simulink library "StIsPosChkLib"  (R2018b)
settings: Solver=VariableStepAuto  StartTime=0.0  StopTime=10.0  RelTol=1e-3
libraries: $bdroot x2, simulink x1
settings Model: Creator=sn2xws  LastModifiedBy=sn2xws

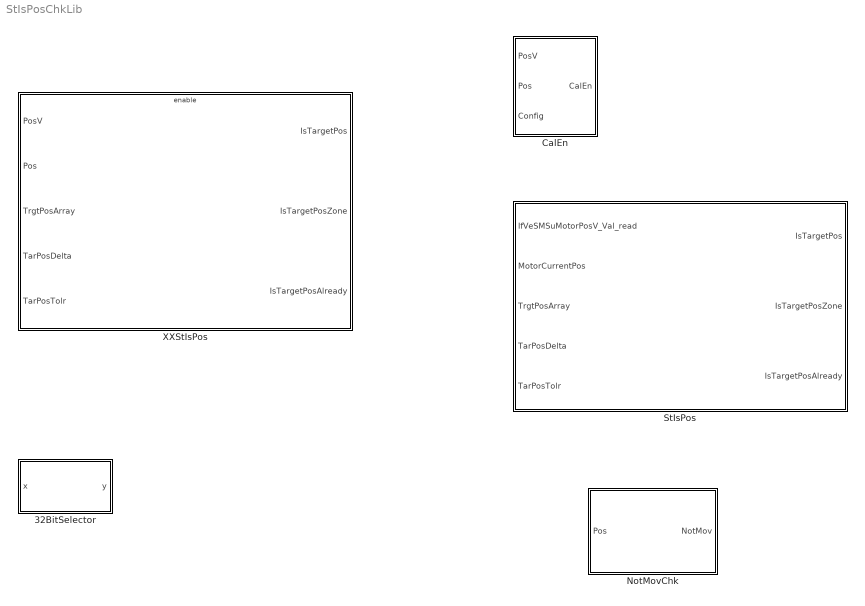
== system StIsPosChkLib ==
  32BitSelector : Subsystem  mask(32 Bit Selector){BitNum=1}
      mask prompts: BitNum "Select Bit Number"
      mask help: Allows selection of a particular bit (0-31) out of a packed word up to 32 bits long. Output will be true if the bit number selected via the mask parameter is equal to one.
      mask TypeOptions BitNum: 0 | 1 | 2 | 3 | 4 | 5 | 6 | 7 | 8 | 9 | 10 | 11 | 12 | 13 | 14 | 15 | 16 | 17 | 18 | 19 | 20 | 21 | 22 | 23 | 24 | 25 | 26 | 27 | 28 | 29 | 30 | 31
      mask Display:
      | text(0.5, 0.8,'BIT','horizontalAlignment','center')
      | text(0.5, 0.5,'SELECTOR','horizontalAlignment','center')
      | text(0.5, 0.2,['-- Bit ',char(get_param(gcb,'BitNum')),' --'],'horizontalAlignment','center')
  CalEn : Subsystem
  NotMovChk : Subsystem
  StIsPos : Subsystem
  XXStIsPos : Subsystem

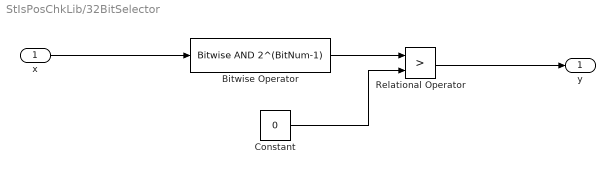
== system StIsPosChkLib/32BitSelector ==
  x : Inport
  Bitwise Operator : simulink/Logic and Bit Operations/Bitwise Operator  logicop=AND  UseBitMask=on  BitMask=2^(BitNum-1)  BitMaskRealWorld=Stored Integer
  Constant : Constant  Value=0  OutDataTypeStr=uint32
  Relational Operator : RelationalOperator  Operator=>  OutDataTypeStr=boolean  RndMeth=Simplest
  y : Outport
  wires:
  Bitwise Operator/1 -> Relational Operator/1
  x/1 -> Bitwise Operator/1
  Constant/1 -> Relational Operator/2
  Relational Operator/1 -> y/1

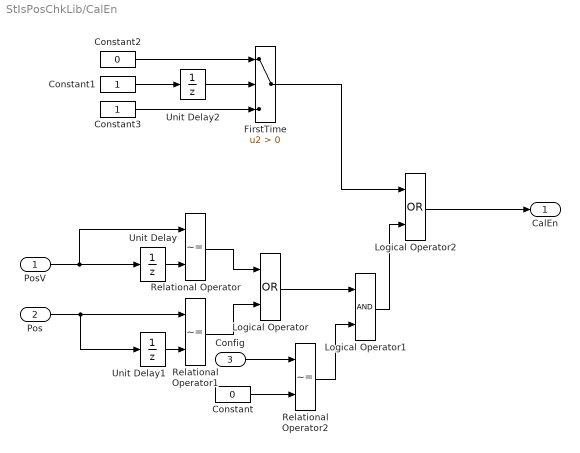
== system StIsPosChkLib/CalEn ==
  PosV : Inport
  Pos : Inport  Port=2
  Config : Inport  Port=3
  Constant : Constant  Value=0  OutDataTypeStr=uint8
  Constant1 : Constant  OutDataTypeStr=boolean
  Constant2 : Constant  Value=0  OutDataTypeStr=boolean
  Constant3 : Constant  OutDataTypeStr=boolean
  FirstTime : Switch  Criteria=u2 > Threshold
  Logical Operator : Logic  Operator=OR  AllPortsSameDT=off  OutDataTypeStr=boolean
  Logical Operator1 : Logic  AllPortsSameDT=off  OutDataTypeStr=boolean
  Logical Operator2 : Logic  Operator=OR  AllPortsSameDT=off  OutDataTypeStr=boolean
  Relational Operator : RelationalOperator  Operator=~=  OutDataTypeStr=boolean  RndMeth=Simplest
  Relational Operator1 : RelationalOperator  Operator=~=  OutDataTypeStr=boolean  RndMeth=Simplest
  Relational Operator2 : RelationalOperator  Operator=~=  OutDataTypeStr=boolean  RndMeth=Simplest
  Unit Delay : UnitDelay  SampleTime=-1
  Unit Delay1 : UnitDelay  SampleTime=-1
  Unit Delay2 : UnitDelay  SampleTime=-1
  CalEn : Outport
  wires:
  Logical Operator/1 -> Logical Operator1/1
  Relational Operator1/1 -> Logical Operator/2
  Unit Delay1/1 -> Relational Operator1/2
  Pos/1 -> Relational Operator1/1, Unit Delay1/1
  Relational Operator/1 -> Logical Operator/1
  Unit Delay/1 -> Relational Operator/2
  PosV/1 -> Unit Delay/1, Relational Operator/1
  Relational Operator2/1 -> Logical Operator1/2
  Config/1 -> Relational Operator2/1
  Constant/1 -> Relational Operator2/2
  Logical Operator1/1 -> Logical Operator2/2
  Logical Operator2/1 -> CalEn/1
  FirstTime/1 -> Logical Operator2/1
  Constant1/1 -> Unit Delay2/1
  Unit Delay2/1 -> FirstTime/2
  Constant2/1 -> FirstTime/1
  Constant3/1 -> FirstTime/3

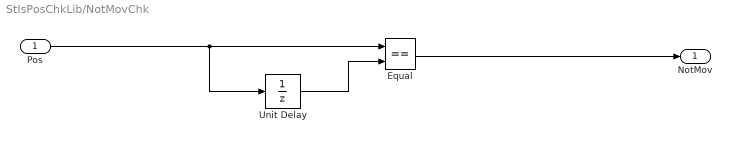
== system StIsPosChkLib/NotMovChk ==
  Pos : Inport
  Equal : RelationalOperator  Operator===  OutDataTypeStr=boolean  RndMeth=Simplest
  Unit Delay : UnitDelay  SampleTime=-1
  NotMov : Outport
  wires:
  Equal/1 -> NotMov/1
  Pos/1 -> Equal/1, Unit Delay/1
  Unit Delay/1 -> Equal/2

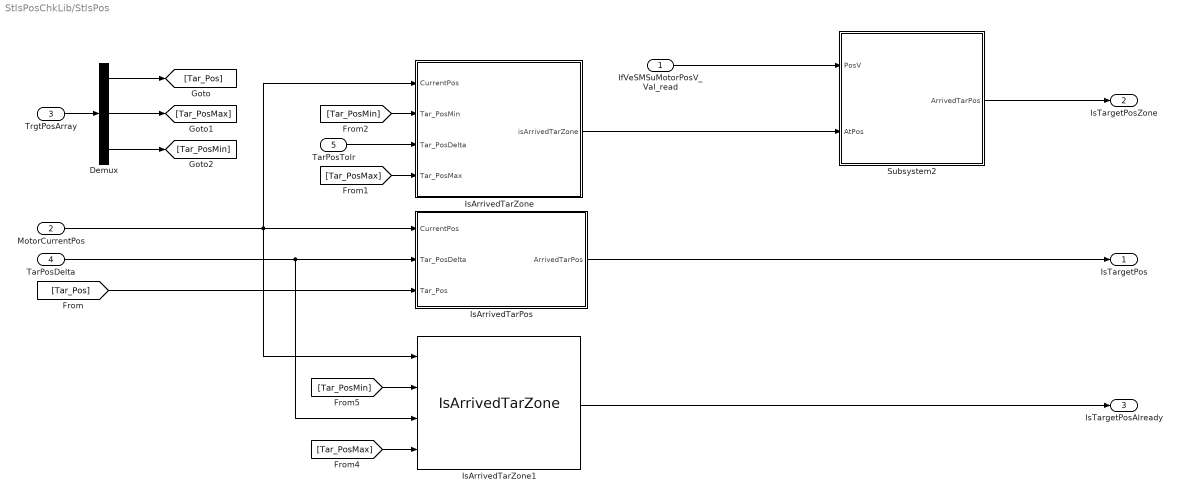
== system StIsPosChkLib/StIsPos ==
  IfVeSMSuMotorPosV_Val_read : Inport
  MotorCurrentPos : Inport  Port=2
  TrgtPosArray : Inport  Port=3
  TarPosDelta : Inport  Port=4
  TarPosTolr : Inport  Port=5
  Demux : Demux  Outputs=3
  IsArrivedTarPos : Subsystem
  IsArrivedTarZone : Subsystem
  IsArrivedTarZone1 : $bdroot/StIsPos/IsArrivedTarZone  SystemSampleTime=-1
  Subsystem2 : Subsystem
  IsTargetPos : Outport
      settings: EnsureOutportIsVirtual=on
  IsTargetPosZone : Outport  Port=2
      settings: EnsureOutportIsVirtual=on
  IsTargetPosAlready : Outport  Port=3
      settings: EnsureOutportIsVirtual=on
  wires:
  MotorCurrentPos/1 -> IsArrivedTarZone/1(CurrentPos), IsArrivedTarZone1/1, IsArrivedTarPos/1(CurrentPos)
  IsArrivedTarPos/1(ArrivedTarPos) -> IsTargetPos/1
  Subsystem2/1(ArrivedTarPos) -> IsTargetPosZone/1
  IfVeSMSuMotorPosV_Val_read/1 -> Subsystem2/1(PosV)
  IsArrivedTarZone/1(isArrivedTarZone) -> Subsystem2/2(AtPos)
  TrgtPosArray/1 -> Demux/1
  Demux/1 -> [Tar_Pos]
  Demux/2 -> [Tar_PosMax]
  Demux/3 -> [Tar_PosMin]
  [Tar_Pos] -> IsArrivedTarPos/3(Tar_Pos)
  [Tar_PosMax] -> IsArrivedTarZone/4(Tar_PosMax)
  [Tar_PosMin] -> IsArrivedTarZone/2(Tar_PosMin)
  [Tar_PosMax] -> IsArrivedTarZone1/4
  [Tar_PosMin] -> IsArrivedTarZone1/2
  TarPosDelta/1 -> IsArrivedTarZone1/3, IsArrivedTarPos/2(Tar_PosDelta)
  TarPosTolr/1 -> IsArrivedTarZone/3(Tar_PosDelta)
  IsArrivedTarZone1/1 -> IsTargetPosAlready/1

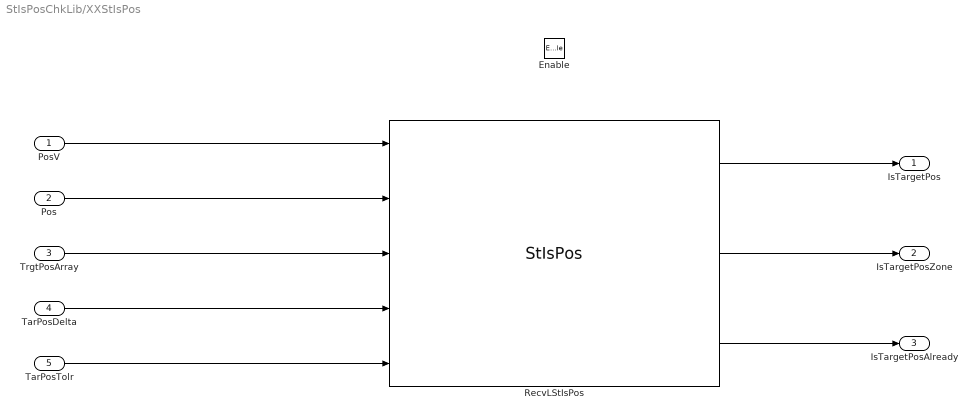
== system StIsPosChkLib/XXStIsPos ==
  PosV : Inport
  Pos : Inport  Port=2
  TrgtPosArray : Inport  Port=3
  TarPosDelta : Inport  Port=4
  TarPosTolr : Inport  Port=5
  Enable : EnablePort
  RecvLStIsPos : $bdroot/StIsPos  SystemSampleTime=-1
  IsTargetPos : Outport
  IsTargetPosZone : Outport  Port=2
  IsTargetPosAlready : Outport  Port=3
  wires:
  TarPosTolr/1 -> RecvLStIsPos/5
  TrgtPosArray/1 -> RecvLStIsPos/3
  PosV/1 -> RecvLStIsPos/1
  TarPosDelta/1 -> RecvLStIsPos/4
  Pos/1 -> RecvLStIsPos/2
  RecvLStIsPos/1 -> IsTargetPos/1
  RecvLStIsPos/3 -> IsTargetPosAlready/1
  RecvLStIsPos/2 -> IsTargetPosZone/1

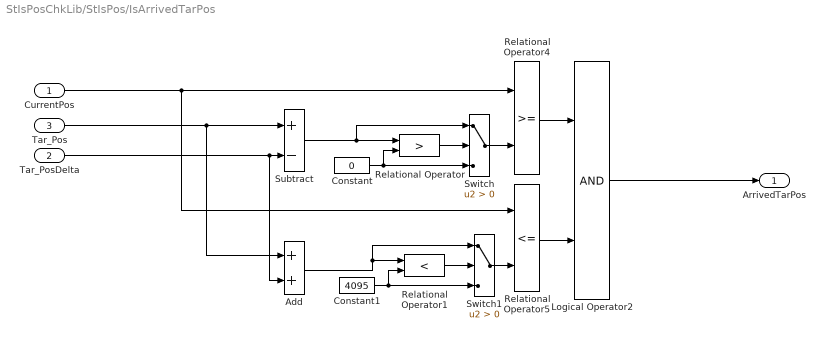
== system StIsPosChkLib/StIsPos/IsArrivedTarPos ==
  CurrentPos : Inport
  Tar_PosDelta : Inport  Port=2
  Tar_Pos : Inport  Port=3
  Add : Sum
  Constant : Constant  Value=0  OutDataTypeStr=uint16
  Constant1 : Constant  Value=4095  OutDataTypeStr=uint16
  Logical Operator2 : Logic  AllPortsSameDT=off  OutDataTypeStr=boolean
  Relational Operator : RelationalOperator  Operator=>  OutDataTypeStr=boolean  RndMeth=Simplest
  Relational Operator1 : RelationalOperator  Operator=<  OutDataTypeStr=boolean  RndMeth=Simplest
  Relational Operator4 : RelationalOperator  OutDataTypeStr=boolean  RndMeth=Simplest
  Relational Operator5 : RelationalOperator  Operator=<=  OutDataTypeStr=boolean  RndMeth=Simplest
  Subtract : Sum  Inputs=+-  OutDataTypeStr=int16
  Switch : Switch  Criteria=u2 > Threshold
  Switch1 : Switch  Criteria=u2 > Threshold
  ArrivedTarPos : Outport
  wires:
  Relational Operator5/1 -> Logical Operator2/2
  Tar_Pos/1 -> Add/1, Subtract/1
  Relational Operator4/1 -> Logical Operator2/1
  Tar_PosDelta/1 -> Add/2, Subtract/2
  Switch/1 -> Relational Operator4/2
  CurrentPos/1 -> Relational Operator4/1, Relational Operator5/1
  Logical Operator2/1 -> ArrivedTarPos/1
  Subtract/1 -> Switch/1, Relational Operator/1
  Relational Operator/1 -> Switch/2
  Constant/1 -> Relational Operator/2, Switch/3
  Add/1 -> Switch1/1, Relational Operator1/1
  Constant1/1 -> Relational Operator1/2, Switch1/3
  Switch1/1 -> Relational Operator5/2
  Relational Operator1/1 -> Switch1/2

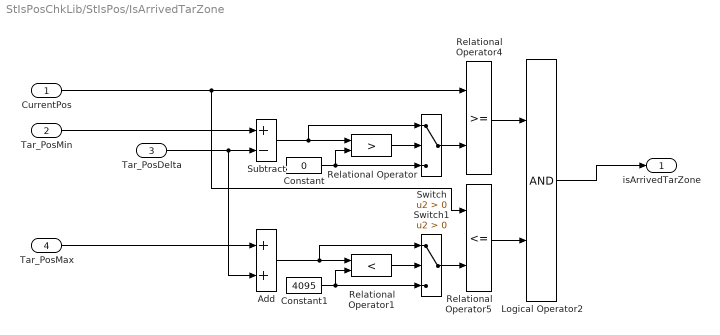
== system StIsPosChkLib/StIsPos/IsArrivedTarZone ==
  CurrentPos : Inport
  Tar_PosMin : Inport  Port=2
  Tar_PosDelta : Inport  Port=3
  Tar_PosMax : Inport  Port=4
  Add : Sum
  Constant : Constant  Value=0  OutDataTypeStr=uint16
  Constant1 : Constant  Value=4095  OutDataTypeStr=uint16
  Logical Operator2 : Logic  AllPortsSameDT=off  OutDataTypeStr=boolean
  Relational Operator : RelationalOperator  Operator=>  OutDataTypeStr=boolean  RndMeth=Simplest
  Relational Operator1 : RelationalOperator  Operator=<  OutDataTypeStr=boolean  RndMeth=Simplest
  Relational Operator4 : RelationalOperator  OutDataTypeStr=boolean  RndMeth=Simplest
  Relational Operator5 : RelationalOperator  Operator=<=  OutDataTypeStr=boolean  RndMeth=Simplest
  Subtract : Sum  Inputs=+-  OutDataTypeStr=int16
  Switch : Switch  Criteria=u2 > Threshold
  Switch1 : Switch  Criteria=u2 > Threshold
  isArrivedTarZone : Outport
  wires:
  Tar_PosDelta/1 -> Subtract/2, Add/2
  Add/1 -> Switch1/1, Relational Operator1/1
  Switch1/1 -> Relational Operator5/2
  CurrentPos/1 -> Relational Operator4/1, Relational Operator5/1
  Tar_PosMin/1 -> Subtract/1
  Switch/1 -> Relational Operator4/2
  Logical Operator2/1 -> isArrivedTarZone/1
  Relational Operator5/1 -> Logical Operator2/2
  Tar_PosMax/1 -> Add/1
  Relational Operator4/1 -> Logical Operator2/1
  Subtract/1 -> Switch/1, Relational Operator/1
  Constant/1 -> Relational Operator/2, Switch/3
  Relational Operator/1 -> Switch/2
  Relational Operator1/1 -> Switch1/2
  Constant1/1 -> Relational Operator1/2, Switch1/3

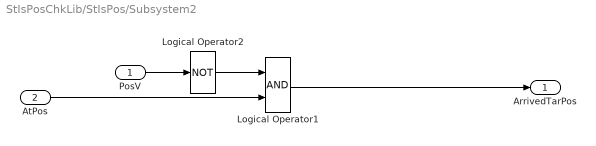
== system StIsPosChkLib/StIsPos/Subsystem2 ==
  PosV : Inport
  AtPos : Inport  Port=2
  Logical Operator1 : Logic  AllPortsSameDT=off  OutDataTypeStr=boolean
  Logical Operator2 : Logic  Operator=NOT  AllPortsSameDT=off  OutDataTypeStr=boolean
  ArrivedTarPos : Outport
  wires:
  Logical Operator2/1 -> Logical Operator1/1
  PosV/1 -> Logical Operator2/1
  AtPos/1 -> Logical Operator1/2
  Logical Operator1/1 -> ArrivedTarPos/1
